simulink model "clase4"  (R2018a)
settings: Solver=VariableStepAuto  StartTime=0.0  StopTime=10.0  RelTol=1e-3
libraries: cstblocks x1
settings Model: Creator=napoleon  LastModifiedBy=napoleon

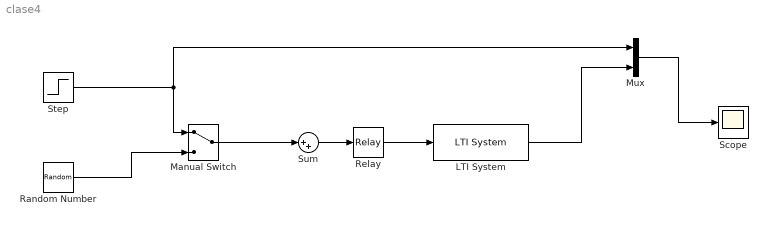
== system clase4 ==
  LTI System : cstblocks/LTI System  sys=tf(1,[1 1])  IC=[]
  Manual Switch : ManualSwitch
  Mux : Mux  Inputs=2
  Random Number : RandomNumber  SampleTime=0.1
  Relay : Relay
  Scope : Scope
  Step : Step  SampleTime=0
  Sum : Sum  Inputs=|++
  wires:
  Step/1 -> Manual Switch/1, Mux/1
  Random Number/1 -> Manual Switch/2
  Manual Switch/1 -> Sum/1
  Sum/1 -> Relay/1
  Mux/1 -> Scope/1
  Relay/1 -> LTI System/1
  LTI System/1 -> Mux/2
